simulink model "thyristor"  (R2018a)
settings: Solver=VariableStepAuto  StartTime=2  StopTime=5  RelTol=1e-3
libraries: powerlib x10
settings Model: Creator=ROG  LastModifiedBy=furkan

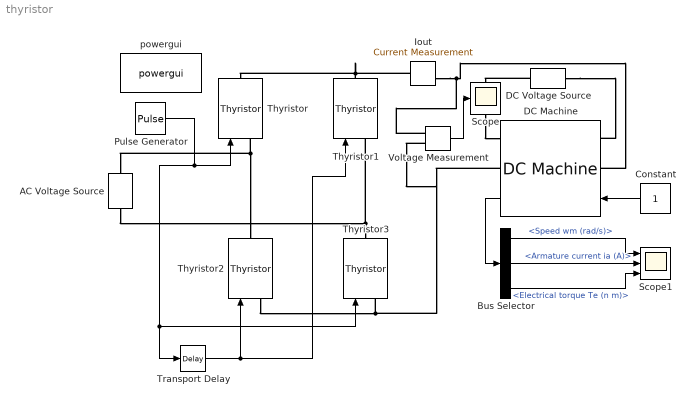
== system thyristor ==
  AC Voltage Source : powerlib/Electrical Sources/AC Voltage Source  Amplitude=230*sqrt(2)  Phase=0  Frequency=50  SampleTime=0  Measurements=None  BusType=swing  Pref=10e3  Qref=0  Qmin=-inf  Qmax=+inf
  Bus Selector : BusSelector  OutputSignals=Speed wm (rad/s),Armature current ia (A),Electrical torque Te (n m)
  Constant : Constant
  DC Machine : powerlib/Machines/DC Machine  PresetModel=No  MechanicalLoad=Torque TL  FieldType=Wound  ShowDetailedParameters=on  MeasurementBus=off  RLa="[ 0.8  0.0125]"  RLf="[ 8260  6.4]"  Laf=5  MachineConstant=Torque constant (N.m/A)  Ke=1.8  Kt=1.8  J=1  Bm=0  Tf=0  w0=50  Ifinit=1  TsPowergui=0  TsBlock=-1
  DC Voltage Source : powerlib/Electrical Sources/DC Voltage Source  Amplitude=100  Measurements=None
  Iout : powerlib/Measurements/Current Measurement  PhasorSimulation=off  OutputType=Complex  PSBequivalent=0
  Pulse Generator : DiscretePulseGenerator  PulseType=Time based  Amplitude=5  Period=0.02  PulseWidth=5  PhaseDelay=(0*0.02)/360
  Scope : Scope
  Scope1 : Scope  NumInputPorts=3
  Thyristor{,1..3} (4 alike) : powerlib/Power Electronics/Thyristor  Ron=0.001  Lon=0  Vf=0  IC=0  Rs=500  Cs=250e-9  Measurements=off
  Transport Delay : TransportDelay  DelayTime=0.01
  Voltage Measurement : powerlib/Measurements/Voltage Measurement  PhasorSimulation=off  OutputType=Complex  PSBequivalent=0
  powergui : powerlib/powergui  Priority=1  SimulationMode=Discrete  SampleTime=5e-6  frequency=60  Iterations=50  frequencyindice=0  Pbase=100e6  ErrMax=1e-4  UnitsV=kV  UnitsW=MW  buscounter=0  FunctionMessages=off  echomessages=off  EnableUseOfTLC=off  CurrentSourceSwitches=off  DisableSnubberDevices=off  DisableRonSwitches=off  DisableVfSwitches=off  DisplayEquations=off  SolverType=Tustin/Backward Euler (TBE)  Interpol=off  ExternalGateDelay=off  methode=off  Ts=100  x0status=blocks  SPID=off  SwTol=0  HookPort=off  RestoreLinks=warning  ResistiveCurrentMeasurement=off  Frange=[0:2:500]  Ylog=off  Xlog=on  ShowGrid=off  save=off  variable=ZData  structure=InputCurrent  ZoomFFT=off  StartTime=2.5  cycles=100  DisplayStyle=2  fundamental=50  FreqAxis=off  MaxFrequency=1000  frequencyindicesteady=1  RmsSteady=1  display=off
  wires:
  Pulse Generator/1 -> Thyristor/1, Thyristor3/1, Transport Delay/1
  Transport Delay/1 -> Thyristor1/1, Thyristor2/1
  Bus Selector/2 -> Scope1/2  "<Armature current ia (A)>"
  Constant/1 -> DC Machine/1
  DC Machine/1 -> Bus Selector/1
  Bus Selector/1 -> Scope1/1  "<Speed wm (rad/s)>"
  Bus Selector/3 -> Scope1/3  "<Electrical torque Te (n m)>"
  Voltage Measurement/1 -> Scope/1
  connections:
  Iout/RConn1 -- Voltage Measurement/LConn1 -- DC Machine/LConn1
  Thyristor1/RConn1 -- Iout/LConn1 -- Thyristor/RConn1
  AC Voltage Source/LConn1 -- Thyristor1/LConn1 -- Thyristor3/RConn1
  Thyristor2/LConn1 -- Voltage Measurement/LConn2 -- DC Machine/RConn1 -- Thyristor3/LConn1
  Thyristor/LConn1 -- AC Voltage Source/RConn1 -- Thyristor2/RConn1
  DC Voltage Source/RConn1 -- DC Machine/LConn2
  DC Voltage Source/LConn1 -- DC Machine/RConn2
